simulink model "Sim2"  (R2022a)
settings: Solver=ode4  StartTime=0.0  StopTime=100  FixedStep=0.005  RelTol=1e-3
libraries: slpidlib x1
settings Model: Creator=81909  LastModifiedBy=81909

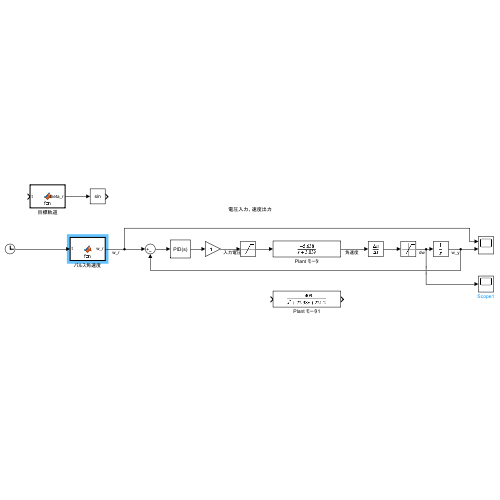
[thumbnail: Simulink's stored preview of the top-level diagram]
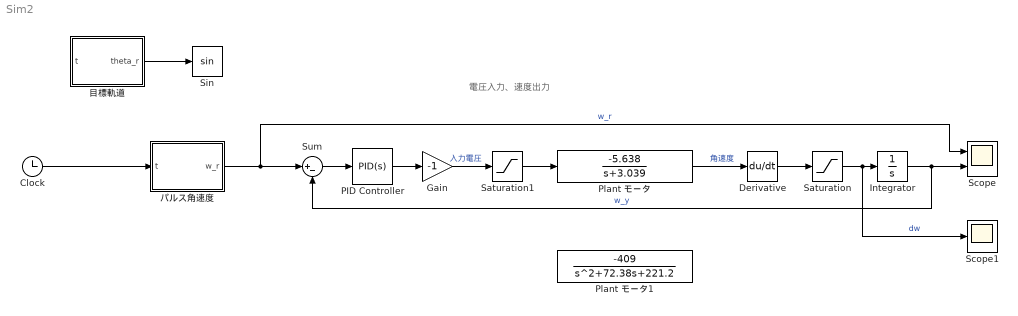
== system Sim2 ==
  note: 電圧入力、速度出力
  Clock : Clock
  Derivative : Derivative
  Gain : Gain  Gain=-1
  Integrator : Integrator
  PID Controller : slpidlib/PID Controller  Controller=PID  Form=Parallel  TimeDomain=Continuous-time  UseExternalTs=off  SampleTime=-1  IntegratorMethod=Forward Euler  FilterMethod=Forward Euler  ControllerParametersSource=internal  P=1  I=0.5719  UseKiTs=off  D=1  N=100  UseFilter=on  TunerSelectOption=Frequency Response Based  InitialConditionSource=internal  InitialConditionForIntegrator=0  InitialConditionForFilter=0  DifferentiatorICPrevScaledInput=0  ExternalReset=none  TrackingMode=off  Kt=1  LimitOutput=off  SatLimitsSource=internal  UpperSaturationLimit=inf  LowerSaturationLimit=-inf  LinearizeAsGain=on  AntiWindupMode=none  Kb=1  POutMin=[]  POutMax=[]  IOutMin=[]  IOutMax=[]  DOutMin=[]  DOutMax=[]  NOutMin=[]  NOutMax=[]  SumOutMin=[]  SumOutMax=[]  SaturationOutMin=[]  SaturationOutMax=[]  PParamMin=[]  PParamMax=[]  IParamMin=[]  IParamMax=[]  DParamMin=[]  DParamMax=[]  NParamMin=[]  NParamMax=[]  KbParamMin=[]  KbParamMax=[]  KtParamMin=[]  KtParamMax=[]  KbOutMin=[]  KbOutMax=[]  KtOutMin=[]  KtOutMax=[]  IntegratorOutMin=[]  IntegratorOutMax=[]  FilterOutMin=[]  FilterOutMax=[]  SumI1OutMin=[]  SumI1OutMax=[]  SumI2OutMin=[]  SumI2OutMax=[]  SumI3OutMin=[]  SumI3OutMax=[]  SumI4OutMin=[]  SumI4OutMax=[]  SumDOutMin=[]  SumDOutMax=[]  DifferentiatorOutMin=[]  DifferentiatorOutMax=[]  FilterDiffOutCoefMin=[]  FilterDiffOutCoefMax=[]  ReciprocalOutMin=[]  ReciprocalOutMax=[]  SumDenOutMin=[]  SumDenOutMax=[]  SumNumOutMin=[]  SumNumOutMax=[]  DivideOutMin=[]  DivideOutMax=[]  UdiffTsProdOutMin=[]  UdiffTsProdOutMax=[]  NTsProdOutMin=[]  NTsProdOutMax=[]  UintegralTsProdOutMin=[]  UintegralTsProdOutMax=[]  UngainTsProdOutMin=[]  UngainTsProdOutMax=[]  IntegratorContinuousStateAttributes=''  IntegratorStateMustResolveToSignalObject=off  IntegratorRTWStateStorageClass=Auto  FilterContinuousStateAttributes=''  FilterStateMustResolveToSignalObject=off  FilterRTWStateStorageClass=Auto  ParallelPVariant=InternalParameters  IdealPVariant=Disabled  IVariant=InternalParameters  DVariant=InternalParameters  IntegratorVariant=Continuous  SatVariant=Disabled  AWVariant=Passthrough  PCopyVariant=Disabled  TRVariant=Disabled  FdbkBlocksVariant=Forward  IdealPFdbkVariant=Disabled  SatFdbkVariant=Disabled  DerivativeFilterVariant=ContFilter  NVariant=InternalParameters  NCopyVariant=Disabled  FilterICVariant=InternalICsFilter  IntegratorICVariant=InternalICs  ExternalResetVariant=Disabled  TRSumVariant=Passthrough  SumFdbkVariant=Disabled  SumVariant=Sum_PID  TsampFilterVariant=InternalTs  TsampNgainVariant=Passthrough  TsampIntegralVariant=Passthrough  ExternalSaturationOutDataTypeStr=Inherit: Same as second input  aMode=0
  Plant モータ : TransferFcn  Numerator=[-5.638]  Denominator=[1 3.039]
  Plant モータ1 : TransferFcn  Numerator=[-409]  Denominator=[1 72.38 221.2]
  Saturation : Saturate  UpperLimit=43  LowerLimit=-44.15
  Saturation1 : Saturate  UpperLimit=12  LowerLimit=0
  Scope : Scope  NumInputPorts=2
  Scope1 : Scope
  Sin : Trigonometry
  Sum : Sum  Inputs=|+-
  パルス角速度 : MATLAB Function  TreatAsAtomicUnit=on
  目標軌道 : MATLAB Function  TreatAsAtomicUnit=on
  wires:
  Plant モータ/1 -> Derivative/1  "角速度"
  Derivative/1 -> Saturation/1
  Saturation/1 -> Scope1/1, Integrator/1  "dw"
  Integrator/1 -> Sum/2, Scope/2  "w_y"
  パルス角速度/1(w_r) -> Sum/1, Scope/1  "w_r"
  Clock/1 -> パルス角速度/1(t)
  目標軌道/1(theta_r) -> Sin/1
  PID Controller/1 -> Gain/1
  Sum/1 -> PID Controller/1
  Gain/1 -> Saturation1/1  "入力電圧"
  Saturation1/1 -> Plant モータ/1

== matlab function Sim2/目標軌道 ==
  data: t input; theta_r output
function theta_r = fcn(t)
% 目標軌道をコーディングして、微分器で目標角速度を出す

T = 0.4; % 鍋の周期は0.4sくらい
pi = 3.1415;

theta_r = 2*pi/T*t;

== matlab function Sim2/パルス角速度 ==
  data: t input; w_r output
function w_r = fcn(t)
T = 0.4;

if(rem(t, T) <= 0.3)
    w_r = 0.15;
else
    w_r = 0.5;
end
